simulink model "forno"  (Simulink 10.0)
settings: Solver=ode5  StartTime=0.0  StopTime=3e3  FixedStep=1e-2  RelTol=1e-4  EnableMultiTasking=on
values from neighbouring files (symbols this model uses):
  A = [-(Gc+Gf)/Cf Gc/Cf;Gc/Cc -Gc/Cc]    [s_forno.m]
  B = [1/Cf Gf/Cf;0 0]    [s_forno.m]
  C = eye(2)    [s_forno.m]
  D = zeros(2,2)    [s_forno.m]
libraries: simulink x1
settings Model: Creator=prof. G. Celentano  LastModifiedBy=giuseppericcio  ExtModeTrigMode=oneshot  ExtModeArmWhenConnect=off
settings DataIOCC: SignalLoggingSaveFormat=ModelDataLogs  SignalLoggingName=sigsOut
settings OptimizationCC: BooleanDataType=off  ExpressionDepthLimit=2147483647  InitFltsAndDblsToZero=on
settings DebuggingCC: SaveWithParameterizedLinksMsg=none  SignalResolutionControl=TryResolveAllWithWarning  MultiTaskDSMMsg=warning  MultiTaskCondExecSysMsg=none  FcnCallInpInsideContextMsg=warning  StateNameClashWarn=warning
settings HardwareCC: TargetUnknown=on
settings GRTTargetCC: TargetFcnLib=ansi_tfl_tmw.mat

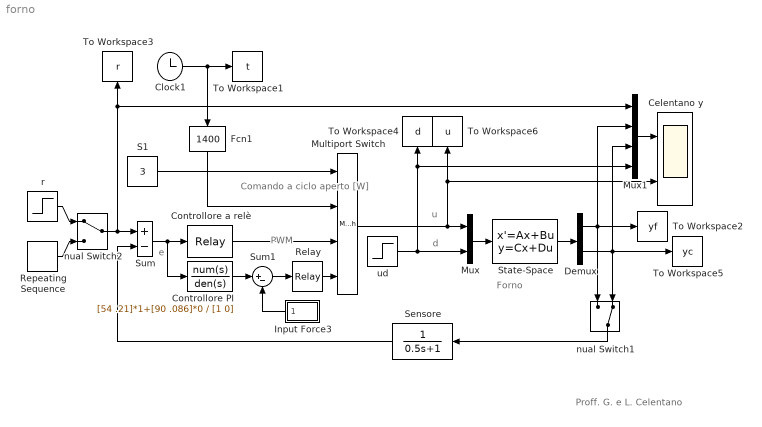
== system forno ==
  note: Comando  a
      |  ciclo aperto [W]
  note: d
  note: u
  note: e
  note: Forno
  note: Proff. G. e L. Celentano
  note: PWM
  Celentano y : Scope  NumInputPorts=2
  Clock1 : Clock
  Controllore PI : TransferFcn  Numerator=[54 .21]*1+[90 .086]*0  Denominator=[1 0]
  Controllore a relè : Relay  OnSwitchValue=5  OffSwitchValue=-5  OnOutputValue=2000
  Demux : Demux  Outputs=2
  Fcn1 : Fcn  Expr=1400
  Input Force3 : Subsystem  mask(Repeating table){rep_seq_t=[0  60], rep_seq_y=[0 2000]}
      mask prompts: rep_seq_t "Time values:"; rep_seq_y "Output values:"
      mask help: Repeating table.
      mask init:
      | period = max(rep_seq_t);
      mask Help: Repeats cycle given in table. Time values should be monotonically increasing.
      mask Display: plot([rep_seq_t,rep_seq_t+period,rep_seq_t+2*period,rep_seq_t(1)+3*period],[rep_seq_y,rep_seq_y,rep_seq_y,rep_seq_y(1)])
  Multiport Switch : MultiPortSwitch  SaturateOnIntegerOverflow=on  InputSameDT=on
  Mux : Mux  Inputs=2
  Mux1 : Mux
  Relay : Relay  OnSwitchValue=0  OffSwitchValue=0  OnOutputValue=2000
  Repeating Sequence : simulink/Sources/Repeating Sequence  rep_seq_t=[0 15*60 70*60 84*60]  rep_seq_y=[10 120 120 10]
  S1 : Constant  Value=3
  Sensore : TransferFcn  Denominator=[0.5 1]
  State-Space : StateSpace  A=A  B=B  C=C  D=D  InitialCondition=[10 10]'
  Sum : Sum  Inputs=+-  SaturateOnIntegerOverflow=on  InputSameDT=on  OutDataTypeStr=Inherit: Same as first input
  Sum1 : Sum  Inputs=|+-  SaturateOnIntegerOverflow=on
  To Workspace1 : ToWorkspace  VariableName=t  SampleTime=-1
  To Workspace2 : ToWorkspace  VariableName=yf  SampleTime=-1
  To Workspace3 : ToWorkspace  VariableName=r  SampleTime=-1
  To Workspace4 : ToWorkspace  VariableName=d  SampleTime=-1
  To Workspace5 : ToWorkspace  VariableName=yc  SampleTime=-1
  To Workspace6 : ToWorkspace  VariableName=u  SampleTime=-1
  nual Switch1 : ManualSwitch  CurrentSetting=0
  nual Switch2 : ManualSwitch
  r : Step  Time=0  After=150  SampleTime=0
  ud : Step  Time=2000  Before=10  After=30  SampleTime=0
  wires:
  Demux/2 -> Mux1/3, To Workspace5/1, nual Switch1/2
  Demux/1 -> To Workspace2/1, Mux1/2, nual Switch1/1
  Clock1/1 -> Fcn1/1, To Workspace1/1
  Multiport Switch/1 -> Mux/1, Celentano y/2, To Workspace6/1
  nual Switch2/1 -> Sum/1, Mux1/1, To Workspace3/1
  Mux1/1 -> Celentano y/1
  ud/1 -> Mux/2, To Workspace4/1, Mux1/4
  Fcn1/1 -> Multiport Switch/2
  S1/1 -> Multiport Switch/1
  Controllore PI/1 -> Sum1/1
  Controllore a relè/1 -> Multiport Switch/3
  Sum/1 -> Controllore a relè/1, Controllore PI/1
  Sensore/1 -> Sum/2
  Mux/1 -> State-Space/1
  State-Space/1 -> Demux/1
  Relay/1 -> Multiport Switch/4
  Input Force3/1(out_1) -> Sum1/2
  Sum1/1 -> Relay/1
  nual Switch1/1 -> Sensore/1
  r/1 -> nual Switch2/1
  Repeating Sequence/1 -> nual Switch2/2

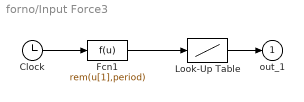
== system forno/Input Force3 ==
  Clock : Clock
  Fcn1 : Fcn  Expr=rem(u[1],period)
  Look-Up Table : Lookup  InputValues=rep_seq_t  Table=rep_seq_y  SaturateOnIntegerOverflow=on
  out_1 : Outport  InitialOutput=0
  wires:
  Fcn1/1 -> Look-Up Table/1
  Clock/1 -> Fcn1/1
  Look-Up Table/1 -> out_1/1
